simulink library "rotationAboutZ"  (R2020a)
settings: Solver=VariableStepAuto  StartTime=0.0  StopTime=10.0  RelTol=1e-3
libraries: sharedutil x1
settings Model: Creator=Ayaz  LastModifiedBy=Ayaz

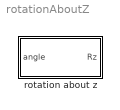
== system rotationAboutZ ==
  rotation about z : Subsystem

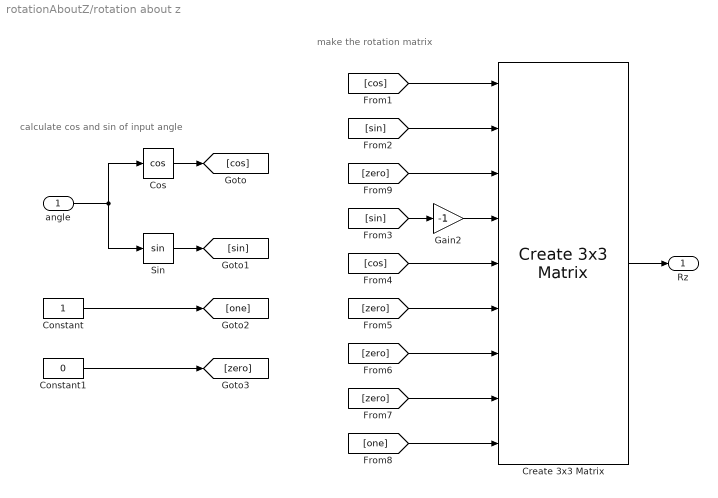
== system rotationAboutZ/rotation about z ==
  note: make the rotation matrix
  note: calculate cos and sin of input angle
  angle : Inport
  Constant : Constant  VectorParams1D=off
  Constant1 : Constant  Value=0  VectorParams1D=off
  Cos : Trigonometry  Operator=cos
  Create 3x3 Matrix : sharedutil/Create 3x3 Matrix  aMode=aMode
      settings: SourceProductBaseCode=AE,PW,MT,VE,VP
  Gain2 : Gain  Gain=-1
  Sin : Trigonometry
  Rz : Outport
  wires:
  angle/1 -> Sin/1, Cos/1
  Cos/1 -> [cos]
  Sin/1 -> [sin]
  Constant/1 -> [one]
  Constant1/1 -> [zero]
  [cos] -> Create 3x3 Matrix/1
  [sin] -> Create 3x3 Matrix/2
  [cos] -> Create 3x3 Matrix/5
  [zero] -> Create 3x3 Matrix/6
  [zero] -> Create 3x3 Matrix/7
  [zero] -> Create 3x3 Matrix/8
  [one] -> Create 3x3 Matrix/9
  Create 3x3 Matrix/1 -> Rz/1
  [zero] -> Create 3x3 Matrix/3
  [sin] -> Gain2/1
  Gain2/1 -> Create 3x3 Matrix/4
